simulink model "LANSwitch"  (R2022b)
settings: Solver=FixedStepAuto  StartTime=0.0  StopTime=10.0  FixedStep=1  RelTol=1e-3
libraries: simulink x34
settings Model: Creator=sadamu  LastModifiedBy=yuzehong
settings OptimizationCC: DefaultParameterBehavior=Inlined  BufferReuse=off  GlobalBufferReuse=off  ExpressionFolding=off  EnableMemcpy=off  PassReuseOutputArgsAs=Individual arguments  NoFixptDivByZeroProtection=on  EfficientFloat2IntCast=on  OptimizeDataStoreBuffers=off  BusAssignmentInplaceUpdate=off  OptimizationLevel=level0  EfficientTunableParamExpr=on
settings DebuggingCC: ParameterTunabilityLossMsg=error  AllowSymbolicDim=off
settings SFSimCC: MATLABDynamicMemAlloc=off
settings RTWCC: Description=Embedded Coder  SystemTargetFile=ert.tlc  GenCodeOnly=on  TemplateMakefile=ert_default_tmf
settings CodeAppCC: GenerateComments=off  IgnoreCustomStorageClasses=off  OperatorAnnotations=on  SimulinkDataObjDesc=on  SFDataObjDesc=on  SimulinkBlockComments=off
settings ERTTargetCC: TargetLangStandard=C99 (ISO)  GenerateSampleERTMain=on  CodeInterfacePackaging=Reusable function  InlinedParameterPlacement=NonHierarchical  ERTCustomFileTemplate=example_file_process.tlc
settings ConfigComp: CovMetricSettings=dcmwe  DVMaxProcessTime=3600  DVTestSuiteOptimization=Auto  DVDetectOutOfBounds=on  DVModelReferenceHarness=on

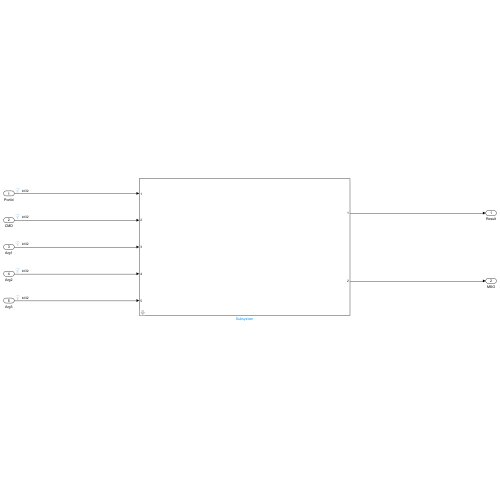
[thumbnail: Simulink's stored preview of the top-level diagram]
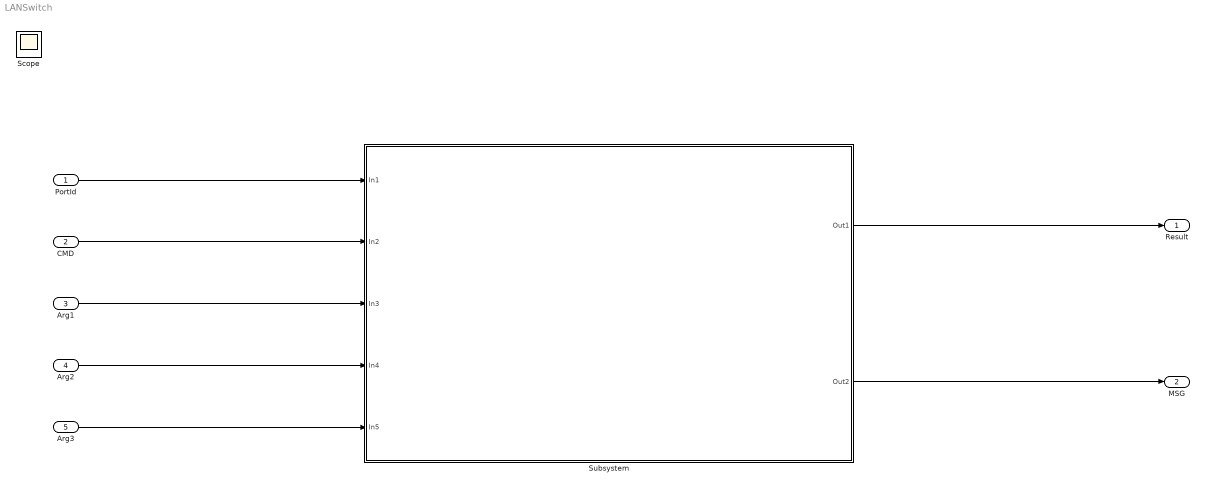
== system LANSwitch ==
  PortId : Inport  OutDataTypeStr=int32
  CMD : Inport  Port=2  OutDataTypeStr=int32
  Arg1 : Inport  Port=3  OutDataTypeStr=int32
  Arg2 : Inport  Port=4  OutDataTypeStr=int32
  Arg3 : Inport  Port=5  OutDataTypeStr=int32
  Subsystem : Subsystem  mask{POOL_SIZE=256}
      mask DialogControl ParameterGroupVar Prompt: 参数
  Result : Outport
  MSG : Outport  Port=2
  Scope : Scope
  wires:
  PortId/1 -> Subsystem/1(In1)
  CMD/1 -> Subsystem/2(In2)
  Arg1/1 -> Subsystem/3(In3)
  Arg2/1 -> Subsystem/4(In4)
  Arg3/1 -> Subsystem/5(In5)
  Subsystem/1(Out1) -> Result/1
  Subsystem/2(Out2) -> MSG/1

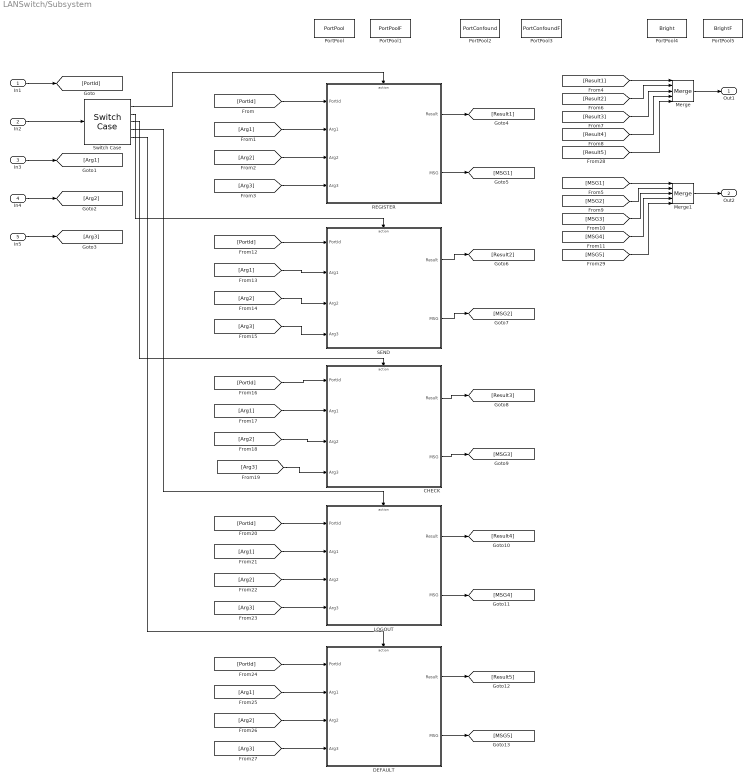
== system LANSwitch/Subsystem ==
  In1 : Inport
  In2 : Inport  Port=2
  In3 : Inport  Port=3
  In4 : Inport  Port=4
  In5 : Inport  Port=5
  CHECK : Subsystem  TreatAsAtomicUnit=on
  DEFAULT : Subsystem  TreatAsAtomicUnit=on
  LOGOUT : Subsystem  TreatAsAtomicUnit=on
  Merge : Merge  Inputs=5
  Merge1 : Merge  Inputs=5
  PortPool : DataStoreMemory  DataStoreName=PortPool  WriteAfterWriteMsg=warning  ShowAdditionalParam=off  OutDataTypeStr=int32  Dimensions=POOL_SIZE
  PortPool1 : DataStoreMemory  DataStoreName=PortPoolF  WriteAfterWriteMsg=warning  ShowAdditionalParam=off  OutDataTypeStr=int32  Dimensions=POOL_SIZE
  PortPool2 : DataStoreMemory  DataStoreName=PortConfound  WriteAfterWriteMsg=warning  ShowAdditionalParam=off  OutDataTypeStr=int32  Dimensions=POOL_SIZE
  PortPool3 : DataStoreMemory  DataStoreName=PortConfoundF  WriteAfterWriteMsg=warning  ShowAdditionalParam=off  OutDataTypeStr=int32  Dimensions=POOL_SIZE
  PortPool4 : DataStoreMemory  DataStoreName=Bright  WriteAfterWriteMsg=warning  ShowAdditionalParam=off  OutDataTypeStr=int32  Dimensions=POOL_SIZE
  PortPool5 : DataStoreMemory  DataStoreName=BrightF  WriteAfterWriteMsg=warning  ShowAdditionalParam=off  OutDataTypeStr=int32  Dimensions=POOL_SIZE
  REGISTER : Subsystem  TreatAsAtomicUnit=on
  SEND : Subsystem  TreatAsAtomicUnit=on
  Switch Case : SwitchCase  CaseConditions={10001, 10002, 10003, 10004}
  Out1 : Outport
  Out2 : Outport  Port=2
  wires:
  DEFAULT/1(Result) -> [Result5]
  REGISTER/1(Result) -> [Result1]
  In2/1 -> Switch Case/1
  [PortId] -> REGISTER/1(PortId)
  [Arg3] -> LOGOUT/4(Arg3)
  CHECK/1(Result) -> [Result3]
  [MSG4] -> Merge1/4
  [Result1] -> Merge/1
  [MSG1] -> Merge1/1
  LOGOUT/2(MSG) -> [MSG4]
  CHECK/2(MSG) -> [MSG3]
  REGISTER/2(MSG) -> [MSG1]
  [Result3] -> Merge/3
  [Arg3] -> SEND/4(Arg3)
  [Arg1] -> REGISTER/2(Arg1)
  [Result5] -> Merge/5
  [Result2] -> Merge/2
  [Result4] -> Merge/4
  [Arg2] -> SEND/3(Arg2)
  [MSG2] -> Merge1/2
  [Arg3] -> DEFAULT/4(Arg3)
  SEND/1(Result) -> [Result2]
  [Arg1] -> SEND/2(Arg1)
  [Arg2] -> REGISTER/3(Arg2)
  [MSG3] -> Merge1/3
  [Arg2] -> DEFAULT/3(Arg2)
  [PortId] -> CHECK/1(PortId)
  Switch Case/2 -> SEND/Action
  In4/1 -> [Arg2]
  Switch Case/5 -> DEFAULT/Action
  SEND/2(MSG) -> [MSG2]
  Switch Case/4 -> LOGOUT/Action
  [Arg2] -> CHECK/3(Arg2)
  [MSG5] -> Merge1/5
  [PortId] -> LOGOUT/1(PortId)
  In5/1 -> [Arg3]
  [Arg3] -> REGISTER/4(Arg3)
  [Arg1] -> DEFAULT/2(Arg1)
  [Arg2] -> LOGOUT/3(Arg2)
  DEFAULT/2(MSG) -> [MSG5]
  Switch Case/3 -> CHECK/Action
  [Arg1] -> CHECK/2(Arg1)
  [PortId] -> SEND/1(PortId)
  In1/1 -> [PortId]
  [Arg3] -> CHECK/4(Arg3)
  LOGOUT/1(Result) -> [Result4]
  Switch Case/1 -> REGISTER/Action
  Merge1/1 -> Out2/1
  [Arg1] -> LOGOUT/2(Arg1)
  [PortId] -> DEFAULT/1(PortId)
  In3/1 -> [Arg1]
  Merge/1 -> Out1/1

== system LANSwitch/Subsystem/CHECK ==
  PortId : Inport
  Arg1 : Inport  Port=2
  Arg2 : Inport  Port=3
  Arg3 : Inport  Port=4
  Action Port : ActionPort  ActionPortLabel=case [ 10003 ]:
  Compare To Constant : simulink/Logic and Bit Operations/Compare To Constant  relop===  const=0  OutDataTypeStr=boolean
  Error : Subsystem  TreatAsAtomicUnit=on
  Handle : Subsystem  TreatAsAtomicUnit=on
  If : If  IfExpression=u1 ~= 0
  Merge : Merge
  Merge1 : Merge
  Result : Outport
  MSG : Outport  Port=2
  wires:
  Arg1/1 -> Handle/2(Arg1)
  Arg2/1 -> Handle/3(Arg2)
  Arg3/1 -> Handle/4(Arg3)
  Merge/1 -> Result/1
  Error/2(MSG) -> Merge1/1
  If/1 -> Error/Action
  If/2 -> Handle/Action
  Merge1/1 -> MSG/1
  PortId/1 -> Handle/1(PortId), Compare To Constant/1
  Error/1(Result) -> Merge/1
  Handle/2(MSG) -> Merge1/2
  Handle/1(Result) -> Merge/2
  Compare To Constant/1 -> If/1

== system LANSwitch/Subsystem/DEFAULT ==
  PortId : Inport
  Arg1 : Inport  Port=2
  Arg2 : Inport  Port=3
  Arg3 : Inport  Port=4
  Action Port : ActionPort  ActionPortLabel=default:
  Constant : Constant  Value=-10002  OutDataTypeStr=int32
  Constant1 : Constant  Value=0  OutDataTypeStr=int32
  Terminator{,1..3} (4 alike) : Terminator
  Result : Outport
  MSG : Outport  Port=2
  wires:
  Constant/1 -> Result/1
  PortId/1 -> Terminator/1
  Arg1/1 -> Terminator1/1
  Arg2/1 -> Terminator2/1
  Arg3/1 -> Terminator3/1
  Constant1/1 -> MSG/1

== system LANSwitch/Subsystem/LOGOUT ==
  PortId : Inport
  Arg1 : Inport  Port=2
  Arg2 : Inport  Port=3
  Arg3 : Inport  Port=4
  Action Port : ActionPort  ActionPortLabel=case [ 10004 ]:
  Compare To Constant : simulink/Logic and Bit Operations/Compare To Constant  relop===  const=0  OutDataTypeStr=boolean
  Error : Subsystem  TreatAsAtomicUnit=on
  Handle : Subsystem  TreatAsAtomicUnit=on
  If : If  IfExpression=u1 ~= 0
  Merge : Merge
  Merge1 : Merge
  Result : Outport
  MSG : Outport  Port=2
  wires:
  PortId/1 -> Handle/1(PortId), Compare To Constant/1
  Compare To Constant/1 -> If/1
  Arg2/1 -> Handle/3(Arg2)
  Error/2(MSG) -> Merge1/1
  Arg1/1 -> Handle/2(Arg1)
  Handle/1(Result) -> Merge/2
  Merge1/1 -> MSG/1
  Error/1(Result) -> Merge/1
  Merge/1 -> Result/1
  If/1 -> Error/Action
  If/2 -> Handle/Action
  Arg3/1 -> Handle/4(Arg3)
  Handle/2(MSG) -> Merge1/2

== system LANSwitch/Subsystem/REGISTER ==
  PortId : Inport
  Arg1 : Inport  Port=2
  Arg2 : Inport  Port=3
  Arg3 : Inport  Port=4
  Action Port : ActionPort  ActionPortLabel=case [ 10001 ]:
  Compare To Constant : simulink/Logic and Bit Operations/Compare To Constant  relop===  const=0  OutDataTypeStr=boolean
  Error : Subsystem  TreatAsAtomicUnit=on
  Handle : Subsystem  TreatAsAtomicUnit=on
  If : If  IfExpression=u1 ~= 0
  Merge : Merge
  Merge1 : Merge
  Result : Outport
  MSG : Outport  Port=2
  wires:
  PortId/1 -> Handle/1(PortId), Compare To Constant/1
  Compare To Constant/1 -> If/1
  If/1 -> Error/Action
  If/2 -> Handle/Action
  Error/1(Result) -> Merge/1
  Handle/1(Result) -> Merge/2
  Merge/1 -> Result/1
  Merge1/1 -> MSG/1
  Error/2(MSG) -> Merge1/1
  Handle/2(MSG) -> Merge1/2
  Arg1/1 -> Handle/2(Arg1)
  Arg2/1 -> Handle/3(Arg2)
  Arg3/1 -> Handle/4(Arg3)

== system LANSwitch/Subsystem/SEND ==
  PortId : Inport
  Arg1 : Inport  Port=2
  Arg2 : Inport  Port=3
  Arg3 : Inport  Port=4
  Action Port : ActionPort  ActionPortLabel=case [ 10002 ]:
  Compare To Constant : simulink/Logic and Bit Operations/Compare To Constant  relop===  const=0  OutDataTypeStr=boolean
  Error : Subsystem  TreatAsAtomicUnit=on
  Handle : Subsystem  TreatAsAtomicUnit=on
  If : If  IfExpression=u1 ~= 0
  Merge : Merge
  Merge1 : Merge
  Result : Outport
  MSG : Outport  Port=2
  wires:
  Arg1/1 -> Handle/2(Arg1)
  Arg2/1 -> Handle/3(Arg2)
  Arg3/1 -> Handle/4(Arg3)
  Merge/1 -> Result/1
  Error/2(MSG) -> Merge1/1
  If/1 -> Error/Action
  If/2 -> Handle/Action
  Merge1/1 -> MSG/1
  PortId/1 -> Handle/1(PortId), Compare To Constant/1
  Error/1(Result) -> Merge/1
  Handle/2(MSG) -> Merge1/2
  Handle/1(Result) -> Merge/2
  Compare To Constant/1 -> If/1

== system LANSwitch/Subsystem/CHECK/Error ==
  Action Port : ActionPort  ActionPortLabel=if(u1 ~= 0)
  Constant : Constant  Value=-10001  OutDataTypeStr=int32
  Constant1 : Constant  Value=0  OutDataTypeStr=int32
  Result : Outport
  MSG : Outport  Port=2
  wires:
  Constant/1 -> Result/1
  Constant1/1 -> MSG/1

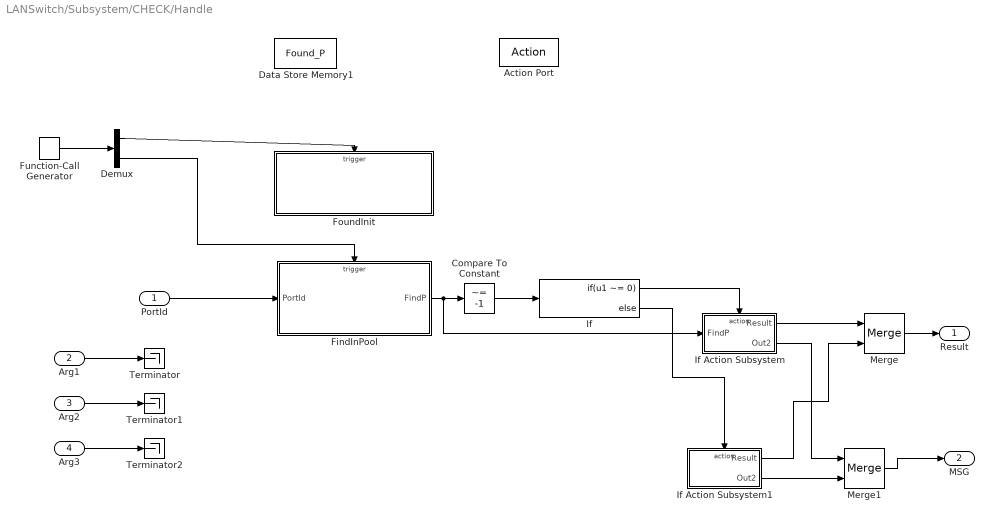
== system LANSwitch/Subsystem/CHECK/Handle ==
  PortId : Inport
  Arg1 : Inport  Port=2
  Arg2 : Inport  Port=3
  Arg3 : Inport  Port=4
  Action Port : ActionPort  ActionPortLabel=else
  Compare To Constant : simulink/Logic and Bit Operations/Compare To Constant  relop=~=  const=-1  OutDataTypeStr=boolean
  Data Store Memory1 : DataStoreMemory  DataStoreName=Found_P  WriteAfterWriteMsg=warning  InitialValue=-1  ShowAdditionalParam=off  OutDataTypeStr=int32
  Demux : Demux  Outputs=2
  FindInPool : Subsystem
  FoundInit : Subsystem
  Function-Call Generator : simulink/Ports & Subsystems/Function-Call Generator  sample_time=1  numberOfIterations=1  DisallowWideOutput=off
  If : If  IfExpression=u1 ~= 0
  If Action Subsystem : Subsystem  TreatAsAtomicUnit=on
  If Action Subsystem1 : Subsystem  TreatAsAtomicUnit=on
  Merge : Merge
  Merge1 : Merge
  Terminator : Terminator
  Terminator1 : Terminator
  Terminator2 : Terminator
  Result : Outport
  MSG : Outport  Port=2
  wires:
  Function-Call Generator/1 -> Demux/1
  Demux/1 -> FoundInit/Trigger
  Demux/2 -> FindInPool/Trigger
  PortId/1 -> FindInPool/1(PortId)
  Arg1/1 -> Terminator/1
  Arg2/1 -> Terminator1/1
  Arg3/1 -> Terminator2/1
  FindInPool/1(FindP) -> If Action Subsystem/1(FindP), Compare To Constant/1
  Compare To Constant/1 -> If/1
  If/1 -> If Action Subsystem/Action
  Merge/1 -> Result/1
  Merge1/1 -> MSG/1
  If Action Subsystem/1(Result) -> Merge/1
  If Action Subsystem/2(Out2) -> Merge1/1
  If Action Subsystem1/1(Result) -> Merge/2
  If Action Subsystem1/2(Out2) -> Merge1/2
  If/2 -> If Action Subsystem1/Action

== system LANSwitch/Subsystem/LOGOUT/Error ==
  Action Port : ActionPort  ActionPortLabel=if(u1 ~= 0)
  Constant : Constant  Value=-10001  OutDataTypeStr=int32
  Constant1 : Constant  Value=0  OutDataTypeStr=int32
  Result : Outport
  MSG : Outport  Port=2
  wires:
  Constant/1 -> Result/1
  Constant1/1 -> MSG/1

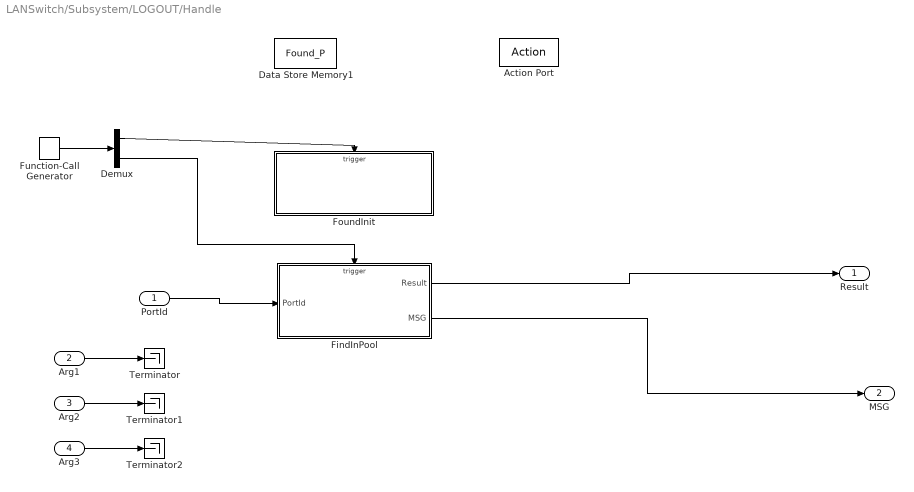
== system LANSwitch/Subsystem/LOGOUT/Handle ==
  PortId : Inport
  Arg1 : Inport  Port=2
  Arg2 : Inport  Port=3
  Arg3 : Inport  Port=4
  Action Port : ActionPort  ActionPortLabel=else
  Data Store Memory1 : DataStoreMemory  DataStoreName=Found_P  WriteAfterWriteMsg=warning  InitialValue=-1  ShowAdditionalParam=off  OutDataTypeStr=int32
  Demux : Demux  Outputs=2
  FindInPool : Subsystem
  FoundInit : Subsystem
  Function-Call Generator : simulink/Ports & Subsystems/Function-Call Generator  sample_time=1  numberOfIterations=1  DisallowWideOutput=off
  Terminator : Terminator
  Terminator1 : Terminator
  Terminator2 : Terminator
  Result : Outport
  MSG : Outport  Port=2
  wires:
  Function-Call Generator/1 -> Demux/1
  Demux/1 -> FoundInit/Trigger
  Demux/2 -> FindInPool/Trigger
  PortId/1 -> FindInPool/1(PortId)
  Arg1/1 -> Terminator/1
  Arg2/1 -> Terminator1/1
  Arg3/1 -> Terminator2/1
  FindInPool/1(Result) -> Result/1
  FindInPool/2(MSG) -> MSG/1

== system LANSwitch/Subsystem/REGISTER/Error ==
  Action Port : ActionPort  ActionPortLabel=if(u1 ~= 0)
  Constant : Constant  Value=-10001  OutDataTypeStr=int32
  Constant1 : Constant  Value=0  OutDataTypeStr=int32
  Result : Outport
  MSG : Outport  Port=2
  wires:
  Constant/1 -> Result/1
  Constant1/1 -> MSG/1

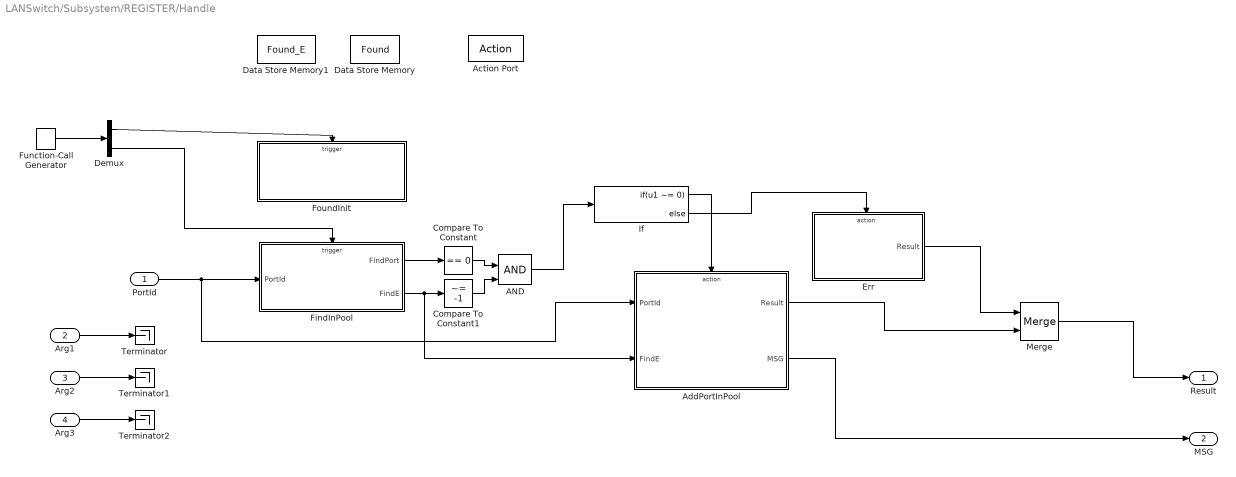
== system LANSwitch/Subsystem/REGISTER/Handle ==
  PortId : Inport
  Arg1 : Inport  Port=2
  Arg2 : Inport  Port=3
  Arg3 : Inport  Port=4
  Action Port : ActionPort  ActionPortLabel=else
  AND : Logic  IconShape=distinctive  AllPortsSameDT=off  OutDataTypeStr=boolean
  AddPortInPool : Subsystem  TreatAsAtomicUnit=on
  Compare To Constant : simulink/Logic and Bit Operations/Compare To Constant  relop===  const=0  OutDataTypeStr=boolean
  Compare To Constant1 : simulink/Logic and Bit Operations/Compare To Constant  relop=~=  const=-1  OutDataTypeStr=boolean
  Data Store Memory : DataStoreMemory  DataStoreName=Found  WriteAfterWriteMsg=warning  ShowAdditionalParam=off  OutDataTypeStr=boolean
  Data Store Memory1 : DataStoreMemory  DataStoreName=Found_E  WriteAfterWriteMsg=warning  InitialValue=-1  ShowAdditionalParam=off  OutDataTypeStr=int32
  Demux : Demux  Outputs=2
  Err : Subsystem  TreatAsAtomicUnit=on
  FindInPool : Subsystem
  FoundInit : Subsystem
  Function-Call Generator : simulink/Ports & Subsystems/Function-Call Generator  sample_time=1  numberOfIterations=1  DisallowWideOutput=off
  If : If  IfExpression=u1 ~= 0
  Merge : Merge
  Terminator : Terminator
  Terminator1 : Terminator
  Terminator2 : Terminator
  Result : Outport
  MSG : Outport  Port=2
  wires:
  Function-Call Generator/1 -> Demux/1
  Demux/1 -> FoundInit/Trigger
  Demux/2 -> FindInPool/Trigger
  PortId/1 -> FindInPool/1(PortId), AddPortInPool/1(PortId)
  AND/1 -> If/1
  Merge/1 -> Result/1
  Err/1(Result) -> Merge/1
  AddPortInPool/1(Result) -> Merge/2
  AddPortInPool/2(MSG) -> MSG/1
  Arg1/1 -> Terminator/1
  Arg2/1 -> Terminator1/1
  Arg3/1 -> Terminator2/1
  FindInPool/1(FindPort) -> Compare To Constant/1
  FindInPool/2(FindE) -> AddPortInPool/2(FindE), Compare To Constant1/1
  Compare To Constant/1 -> AND/1
  Compare To Constant1/1 -> AND/2
  If/2 -> Err/Action
  If/1 -> AddPortInPool/Action

== system LANSwitch/Subsystem/SEND/Error ==
  Action Port : ActionPort  ActionPortLabel=if(u1 ~= 0)
  Constant : Constant  Value=-10001  OutDataTypeStr=int32
  Constant1 : Constant  Value=0  OutDataTypeStr=int32
  Result : Outport
  MSG : Outport  Port=2
  wires:
  Constant/1 -> Result/1
  Constant1/1 -> MSG/1

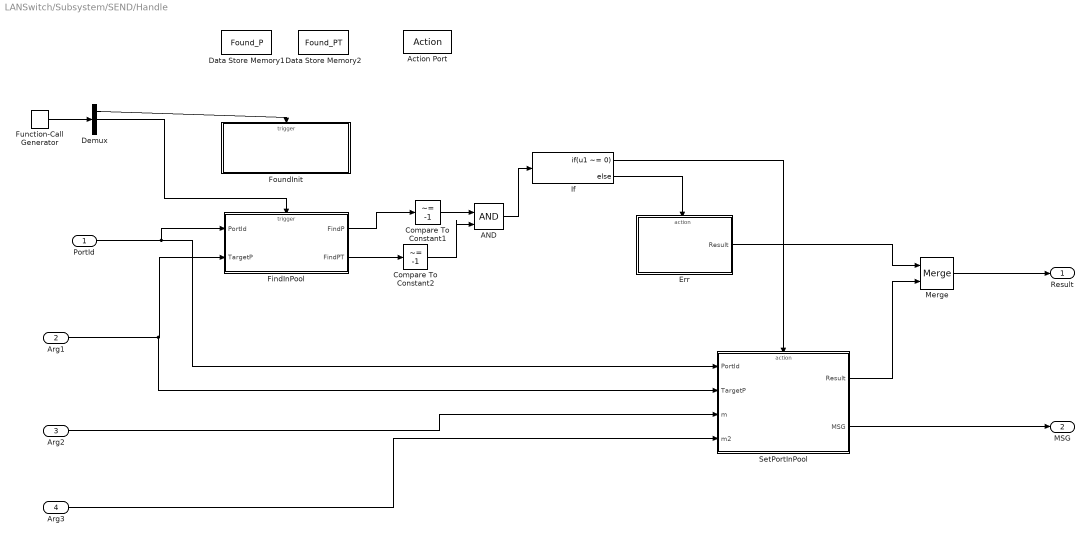
== system LANSwitch/Subsystem/SEND/Handle ==
  PortId : Inport
  Arg1 : Inport  Port=2
  Arg2 : Inport  Port=3
  Arg3 : Inport  Port=4
  Action Port : ActionPort  ActionPortLabel=else
  AND : Logic  IconShape=distinctive  AllPortsSameDT=off  OutDataTypeStr=boolean
  Compare To Constant1 : simulink/Logic and Bit Operations/Compare To Constant  relop=~=  const=-1  OutDataTypeStr=boolean
  Compare To Constant2 : simulink/Logic and Bit Operations/Compare To Constant  relop=~=  const=-1  OutDataTypeStr=boolean
  Data Store Memory1 : DataStoreMemory  DataStoreName=Found_P  WriteAfterWriteMsg=warning  InitialValue=-1  ShowAdditionalParam=off  OutDataTypeStr=int32
  Data Store Memory2 : DataStoreMemory  DataStoreName=Found_PT  WriteAfterWriteMsg=warning  InitialValue=-1  ShowAdditionalParam=off  OutDataTypeStr=int32
  Demux : Demux  Outputs=3
  Err : Subsystem  TreatAsAtomicUnit=on
  FindInPool : Subsystem
  FoundInit : Subsystem
  Function-Call Generator : simulink/Ports & Subsystems/Function-Call Generator  sample_time=1  numberOfIterations=1  DisallowWideOutput=off
  If : If  IfExpression=u1 ~= 0
  Merge : Merge
  SetPortInPool : Subsystem  TreatAsAtomicUnit=on
  Result : Outport
  MSG : Outport  Port=2
  wires:
  Function-Call Generator/1 -> Demux/1
  Demux/1 -> FoundInit/Trigger
  Demux/2 -> FindInPool/Trigger
  PortId/1 -> SetPortInPool/1(PortId), FindInPool/1(PortId)
  If/1 -> SetPortInPool/Action
  Merge/1 -> Result/1
  SetPortInPool/2(MSG) -> MSG/1
  Arg3/1 -> SetPortInPool/4(m2)
  FindInPool/1(FindP) -> Compare To Constant1/1
  Arg1/1 -> SetPortInPool/2(TargetP), FindInPool/2(TargetP)
  FindInPool/2(FindPT) -> Compare To Constant2/1
  Compare To Constant1/1 -> AND/1
  Compare To Constant2/1 -> AND/2
  AND/1 -> If/1
  If/2 -> Err/Action
  SetPortInPool/1(Result) -> Merge/2
  Err/1(Result) -> Merge/1
  Arg2/1 -> SetPortInPool/3(m)

== system LANSwitch/Subsystem/CHECK/Handle/FindInPool ==
  PortId : Inport
  function : TriggerPort  TriggerType=function-call  VariantControl=(inherit)
  FindPortInPool : Subsystem  TreatAsAtomicUnit=on
  FindP : Outport
  wires:
  PortId/1 -> FindPortInPool/1(PortId)
  FindPortInPool/1(Out1) -> FindP/1

== system LANSwitch/Subsystem/CHECK/Handle/FoundInit ==
  function : TriggerPort  TriggerType=function-call  VariantControl=(inherit)
  Constant1 : Constant  Value=-1  OutDataTypeStr=int32
  Data Store Write1 : DataStoreWrite  DataStoreName=Found_P  IndexOptions=Index vector (dialog)  Indices=1  OutputSizes=1
  wires:
  Constant1/1 -> Data Store Write1/1

== system LANSwitch/Subsystem/CHECK/Handle/If Action Subsystem ==
  FindP : Inport
  Action Port : ActionPort  ActionPortLabel=if(u1 ~= 0)
  Constant : Constant  OutDataTypeStr=int32
  Result : Outport
  Out2 : Outport  Port=2
  wires:
  FindP/1 -> Result/1
  Constant/1 -> Out2/1

== system LANSwitch/Subsystem/CHECK/Handle/If Action Subsystem1 ==
  Action Port : ActionPort  ActionPortLabel=else
  Constant : Constant  Value=-1  OutDataTypeStr=int32
  Constant1 : Constant  Value=-1  OutDataTypeStr=int32
  Result : Outport
  Out2 : Outport  Port=2
  wires:
  Constant/1 -> Out2/1
  Constant1/1 -> Result/1

== system LANSwitch/Subsystem/LOGOUT/Handle/FindInPool ==
  PortId : Inport
  function : TriggerPort  TriggerType=function-call  VariantControl=(inherit)
  Compare To Constant1 : simulink/Logic and Bit Operations/Compare To Constant  relop===  const=-1  OutDataTypeStr=uint8
  Err : Subsystem  TreatAsAtomicUnit=on
  FindPortInPool : Subsystem  TreatAsAtomicUnit=on
  If : If  IfExpression=u1 ~= 0
  Merge : Merge
  SetPortInPool : Subsystem  TreatAsAtomicUnit=on
  Result : Outport
  MSG : Outport  Port=2
  wires:
  SetPortInPool/2(MSG) -> MSG/1
  If/1 -> Err/Action
  PortId/1 -> SetPortInPool/1(PortId), FindPortInPool/1(PortId)
  FindPortInPool/1(Out1) -> Compare To Constant1/1
  Err/1(Result) -> Merge/1
  If/2 -> SetPortInPool/Action
  Compare To Constant1/1 -> If/1
  Merge/1 -> Result/1
  SetPortInPool/1(Result) -> Merge/2

== system LANSwitch/Subsystem/LOGOUT/Handle/FoundInit ==
  function : TriggerPort  TriggerType=function-call  VariantControl=(inherit)
  Constant1 : Constant  Value=-1  OutDataTypeStr=int32
  Data Store Write1 : DataStoreWrite  DataStoreName=Found_P  IndexOptions=Index vector (dialog)  Indices=1  OutputSizes=1
  wires:
  Constant1/1 -> Data Store Write1/1

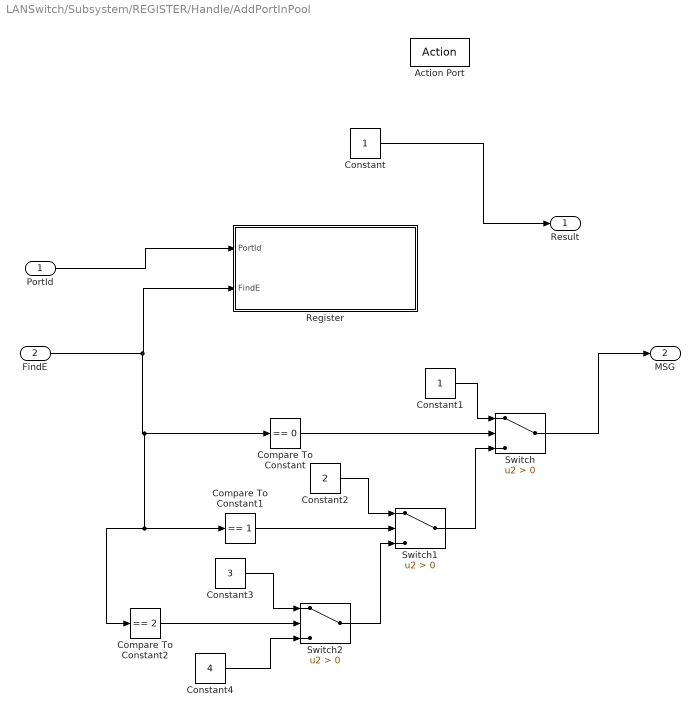
== system LANSwitch/Subsystem/REGISTER/Handle/AddPortInPool ==
  PortId : Inport
  FindE : Inport  Port=2
  Action Port : ActionPort  ActionPortLabel=if(u1 ~= 0)
  Compare To Constant : simulink/Logic and Bit Operations/Compare To Constant  relop===  const=0  OutDataTypeStr=boolean
  Compare To Constant1 : simulink/Logic and Bit Operations/Compare To Constant  relop===  const=1  OutDataTypeStr=boolean
  Compare To Constant2 : simulink/Logic and Bit Operations/Compare To Constant  relop===  const=2  OutDataTypeStr=boolean
  Constant : Constant  OutDataTypeStr=int32
  Constant1 : Constant  OutDataTypeStr=int32
  Constant2 : Constant  Value=2  OutDataTypeStr=int32
  Constant3 : Constant  Value=3  OutDataTypeStr=int32
  Constant4 : Constant  Value=4  OutDataTypeStr=int32
  Register : Subsystem  TreatAsAtomicUnit=on
  Switch : Switch  Criteria=u2 > Threshold  SaturateOnIntegerOverflow=off  InputSameDT=off
  Switch1 : Switch  Criteria=u2 > Threshold  SaturateOnIntegerOverflow=off  InputSameDT=off
  Switch2 : Switch  Criteria=u2 > Threshold  SaturateOnIntegerOverflow=off  InputSameDT=off
  Result : Outport
  MSG : Outport  Port=2
  wires:
  PortId/1 -> Register/1(PortId)
  FindE/1 -> Compare To Constant2/1, Compare To Constant1/1, Compare To Constant/1, Register/2(FindE)
  Constant/1 -> Result/1
  Compare To Constant/1 -> Switch/2
  Constant1/1 -> Switch/1
  Constant2/1 -> Switch1/1
  Compare To Constant1/1 -> Switch1/2
  Switch1/1 -> Switch/3
  Compare To Constant2/1 -> Switch2/2
  Switch2/1 -> Switch1/3
  Constant3/1 -> Switch2/1
  Constant4/1 -> Switch2/3
  Switch/1 -> MSG/1

== system LANSwitch/Subsystem/REGISTER/Handle/Err ==
  Action Port : ActionPort  ActionPortLabel=else
  Constant : Constant  Value=-10004  OutDataTypeStr=int32
  Result : Outport
  wires:
  Constant/1 -> Result/1

== system LANSwitch/Subsystem/REGISTER/Handle/FindInPool ==
  PortId : Inport
  function : TriggerPort  TriggerType=function-call  VariantControl=(inherit)
  FindEmptyInPool : Subsystem  TreatAsAtomicUnit=on
  FindPortInPool : Subsystem  TreatAsAtomicUnit=on
  FindPort : Outport
  FindE : Outport  Port=2
  wires:
  FindPortInPool/1(Out1) -> FindPort/1
  PortId/1 -> FindPortInPool/1(PortId)
  FindEmptyInPool/1(Out1) -> FindE/1

== system LANSwitch/Subsystem/REGISTER/Handle/FoundInit ==
  function : TriggerPort  TriggerType=function-call  VariantControl=(inherit)
  Constant : Constant  Value=0  OutDataTypeStr=boolean
  Constant1 : Constant  Value=-1  OutDataTypeStr=int32
  Data Store Write : DataStoreWrite  DataStoreName=Found  IndexOptions=Index vector (dialog)  Indices=1  OutputSizes=1
  Data Store Write1 : DataStoreWrite  DataStoreName=Found_E  IndexOptions=Index vector (dialog)  Indices=1  OutputSizes=1
  wires:
  Constant/1 -> Data Store Write/1
  Constant1/1 -> Data Store Write1/1

== system LANSwitch/Subsystem/SEND/Handle/Err ==
  Action Port : ActionPort  ActionPortLabel=else
  Constant : Constant  Value=-10003  OutDataTypeStr=int32
  Result : Outport
  wires:
  Constant/1 -> Result/1

== system LANSwitch/Subsystem/SEND/Handle/FindInPool ==
  PortId : Inport
  TargetP : Inport  Port=2
  function : TriggerPort  TriggerType=function-call  VariantControl=(inherit)
  FindPortInPool : Subsystem  TreatAsAtomicUnit=on
  FindPortTInPool : Subsystem  TreatAsAtomicUnit=on
  FindP : Outport
  FindPT : Outport  Port=2
  wires:
  PortId/1 -> FindPortInPool/1(PortId)
  FindPortInPool/1(Out1) -> FindP/1
  TargetP/1 -> FindPortTInPool/1(PortId)
  FindPortTInPool/1(Out1) -> FindPT/1

== system LANSwitch/Subsystem/SEND/Handle/FoundInit ==
  function : TriggerPort  TriggerType=function-call  VariantControl=(inherit)
  Constant1 : Constant  Value=-1  OutDataTypeStr=int32
  Constant2 : Constant  Value=-1  OutDataTypeStr=int32
  Data Store Write1 : DataStoreWrite  DataStoreName=Found_P  IndexOptions=Index vector (dialog)  Indices=1  OutputSizes=1
  Data Store Write2 : DataStoreWrite  DataStoreName=Found_PT  IndexOptions=Index vector (dialog)  Indices=1  OutputSizes=1
  wires:
  Constant1/1 -> Data Store Write1/1
  Constant2/1 -> Data Store Write2/1

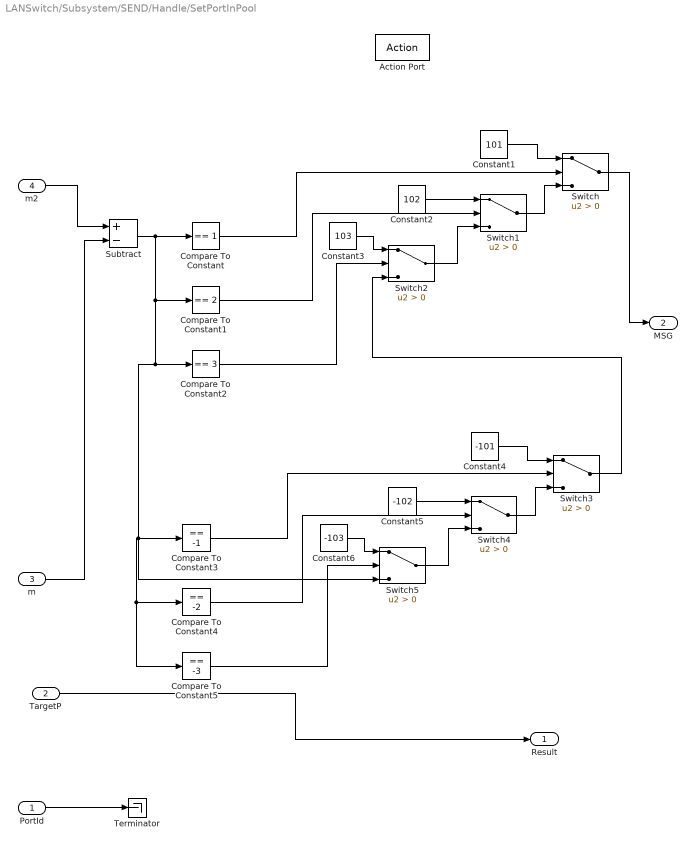
== system LANSwitch/Subsystem/SEND/Handle/SetPortInPool ==
  PortId : Inport
  TargetP : Inport  Port=2
  m : Inport  Port=3
  m2 : Inport  Port=4
  Action Port : ActionPort  ActionPortLabel=if(u1 ~= 0)
  Compare To Constant : simulink/Logic and Bit Operations/Compare To Constant  relop===  const=1  OutDataTypeStr=boolean
  Compare To Constant1 : simulink/Logic and Bit Operations/Compare To Constant  relop===  const=2  OutDataTypeStr=boolean
  Compare To Constant2 : simulink/Logic and Bit Operations/Compare To Constant  relop===  const=3  OutDataTypeStr=boolean
  Compare To Constant3 : simulink/Logic and Bit Operations/Compare To Constant  relop===  const=-1  OutDataTypeStr=boolean
  Compare To Constant4 : simulink/Logic and Bit Operations/Compare To Constant  relop===  const=-2  OutDataTypeStr=boolean
  Compare To Constant5 : simulink/Logic and Bit Operations/Compare To Constant  relop===  const=-3  OutDataTypeStr=boolean
  Constant1 : Constant  Value=101  OutDataTypeStr=int32
  Constant2 : Constant  Value=102  OutDataTypeStr=int32
  Constant3 : Constant  Value=103  OutDataTypeStr=int32
  Constant4 : Constant  Value=-101  OutDataTypeStr=int32
  Constant5 : Constant  Value=-102  OutDataTypeStr=int32
  Constant6 : Constant  Value=-103  OutDataTypeStr=int32
  Subtract : Sum  Inputs=+-
  Switch{,1..5} (6 alike) : Switch  Criteria=u2 > Threshold  SaturateOnIntegerOverflow=off  InputSameDT=off
  Terminator : Terminator
  Result : Outport
  MSG : Outport  Port=2
  wires:
  Compare To Constant/1 -> Switch/2
  Constant1/1 -> Switch/1
  Compare To Constant1/1 -> Switch1/2
  Constant2/1 -> Switch1/1
  Switch1/1 -> Switch/3
  Constant3/1 -> Switch2/1
  Switch2/1 -> Switch1/3
  Compare To Constant2/1 -> Switch2/2
  Constant4/1 -> Switch3/1
  Constant6/1 -> Switch5/1
  Constant5/1 -> Switch4/1
  Compare To Constant4/1 -> Switch4/2
  Compare To Constant5/1 -> Switch5/2
  Switch4/1 -> Switch3/3
  Subtract/1 -> Switch5/3, Compare To Constant5/1, Compare To Constant4/1, Compare To Constant3/1, Compare To Constant2/1, Compare To Constant1/1, Compare To Constant/1
  Compare To Constant3/1 -> Switch3/2
  Switch5/1 -> Switch4/3
  Switch3/1 -> Switch2/3
  Switch/1 -> MSG/1
  m/1 -> Subtract/2
  TargetP/1 -> Result/1
  m2/1 -> Subtract/1
  PortId/1 -> Terminator/1

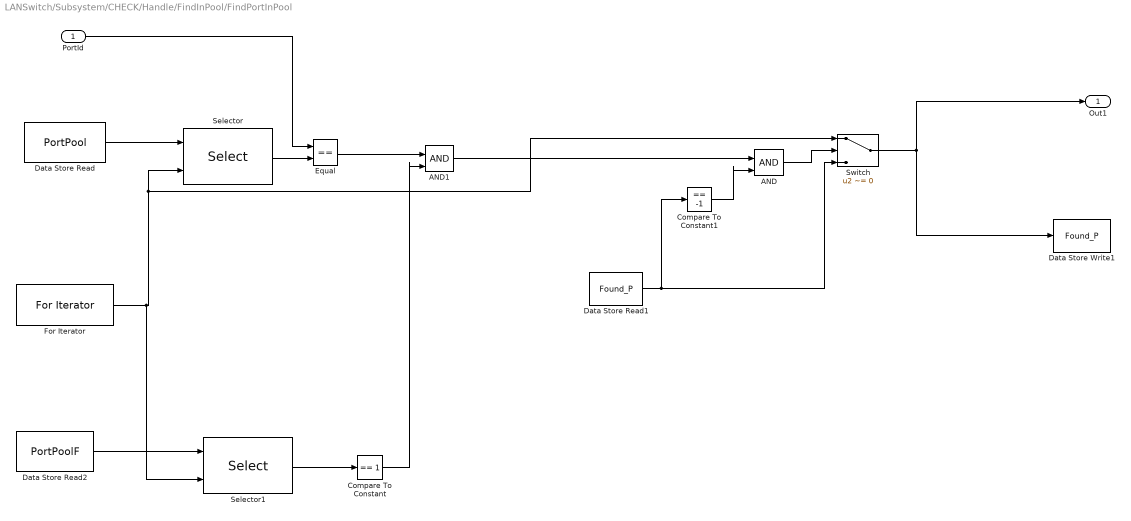
== system LANSwitch/Subsystem/CHECK/Handle/FindInPool/FindPortInPool ==
  PortId : Inport
  AND : Logic  IconShape=distinctive  AllPortsSameDT=off  OutDataTypeStr=boolean
  AND1 : Logic  IconShape=distinctive  AllPortsSameDT=off  OutDataTypeStr=boolean
  Compare To Constant : simulink/Logic and Bit Operations/Compare To Constant  relop===  const=1  OutDataTypeStr=boolean
  Compare To Constant1 : simulink/Logic and Bit Operations/Compare To Constant  relop===  const=-1  OutDataTypeStr=boolean
  Data Store Read : DataStoreRead  DataStoreName=PortPool  IndexOptions=Index vector (dialog)  Indices=1  OutputSizes=1
  Data Store Read1 : DataStoreRead  DataStoreName=Found_P  IndexOptions=Index vector (dialog)  Indices=1  OutputSizes=1
  Data Store Read2 : DataStoreRead  DataStoreName=PortPoolF  IndexOptions=Index vector (dialog)  Indices=1  OutputSizes=1
  Data Store Write1 : DataStoreWrite  DataStoreName=Found_P  IndexOptions=Index vector (dialog)  Indices=1  OutputSizes=1
  Equal : RelationalOperator  Operator===  OutDataTypeStr=boolean  RndMeth=Simplest  InputSameDT=off
  For Iterator : ForIterator  IterationLimit=POOL_SIZE  IndexMode=Zero-based
  Selector : Selector  IndexMode=Zero-based  InputPortWidth=POOL_SIZE  IndexOptions=Index vector (port)  Indices=[1 3]  OutputSizes=1
  Selector1 : Selector  IndexMode=Zero-based  InputPortWidth=POOL_SIZE  IndexOptions=Index vector (port)  Indices=[1 3]  OutputSizes=1
  Switch : Switch  Criteria=u2 ~= 0  SaturateOnIntegerOverflow=off  InputSameDT=off
  Out1 : Outport
  wires:
  Data Store Read/1 -> Selector/1
  Selector/1 -> Equal/2
  Equal/1 -> AND1/1
  Switch/1 -> Data Store Write1/1, Out1/1
  Data Store Read1/1 -> Compare To Constant1/1, Switch/3
  Compare To Constant1/1 -> AND/2
  AND/1 -> Switch/2
  PortId/1 -> Equal/1
  Compare To Constant/1 -> AND1/2
  Data Store Read2/1 -> Selector1/1
  For Iterator/1 -> Selector1/2, Switch/1, Selector/2
  Selector1/1 -> Compare To Constant/1
  AND1/1 -> AND/1

== system LANSwitch/Subsystem/LOGOUT/Handle/FindInPool/Err ==
  Action Port : ActionPort  ActionPortLabel=if(u1 ~= 0)
  Constant : Constant  Value=-10003  OutDataTypeStr=int32
  Result : Outport
  wires:
  Constant/1 -> Result/1

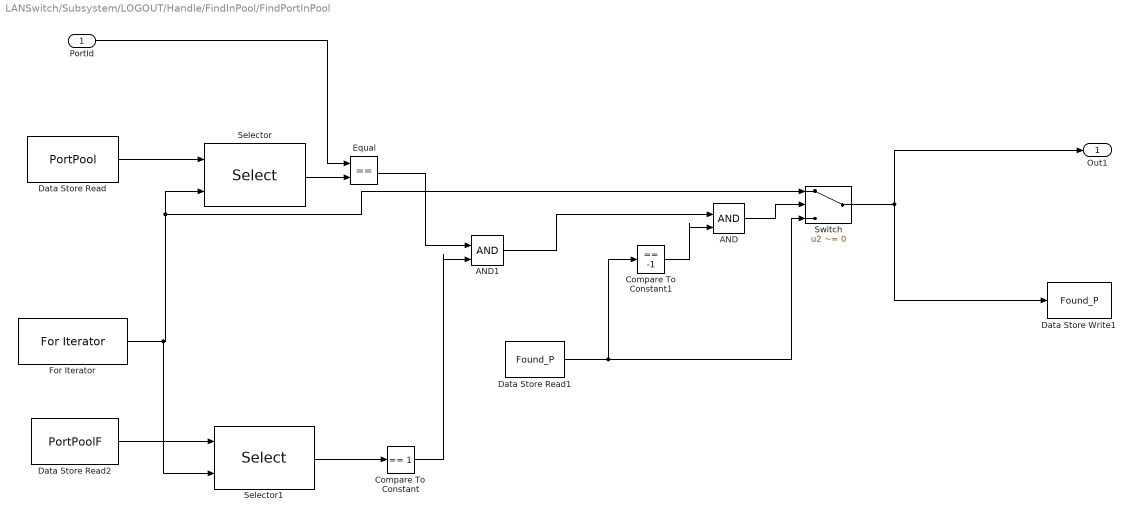
== system LANSwitch/Subsystem/LOGOUT/Handle/FindInPool/FindPortInPool ==
  PortId : Inport
  AND : Logic  IconShape=distinctive  AllPortsSameDT=off  OutDataTypeStr=boolean
  AND1 : Logic  IconShape=distinctive  AllPortsSameDT=off  OutDataTypeStr=boolean
  Compare To Constant : simulink/Logic and Bit Operations/Compare To Constant  relop===  const=1  OutDataTypeStr=boolean
  Compare To Constant1 : simulink/Logic and Bit Operations/Compare To Constant  relop===  const=-1  OutDataTypeStr=boolean
  Data Store Read : DataStoreRead  DataStoreName=PortPool  IndexOptions=Index vector (dialog)  Indices=1  OutputSizes=1
  Data Store Read1 : DataStoreRead  DataStoreName=Found_P  IndexOptions=Index vector (dialog)  Indices=1  OutputSizes=1
  Data Store Read2 : DataStoreRead  DataStoreName=PortPoolF  IndexOptions=Index vector (dialog)  Indices=1  OutputSizes=1
  Data Store Write1 : DataStoreWrite  DataStoreName=Found_P  IndexOptions=Index vector (dialog)  Indices=1  OutputSizes=1
  Equal : RelationalOperator  Operator===  OutDataTypeStr=boolean  RndMeth=Simplest  InputSameDT=off
  For Iterator : ForIterator  IterationLimit=POOL_SIZE  IndexMode=Zero-based
  Selector : Selector  IndexMode=Zero-based  InputPortWidth=POOL_SIZE  IndexOptions=Index vector (port)  Indices=[1 3]  OutputSizes=1
  Selector1 : Selector  IndexMode=Zero-based  InputPortWidth=POOL_SIZE  IndexOptions=Index vector (port)  Indices=[1 3]  OutputSizes=1
  Switch : Switch  Criteria=u2 ~= 0  SaturateOnIntegerOverflow=off  InputSameDT=off
  Out1 : Outport
  wires:
  Data Store Read/1 -> Selector/1
  Selector/1 -> Equal/2
  Equal/1 -> AND1/1
  Switch/1 -> Data Store Write1/1, Out1/1
  Data Store Read1/1 -> Compare To Constant1/1, Switch/3
  Compare To Constant1/1 -> AND/2
  AND/1 -> Switch/2
  PortId/1 -> Equal/1
  Compare To Constant/1 -> AND1/2
  Data Store Read2/1 -> Selector1/1
  For Iterator/1 -> Selector1/2, Switch/1, Selector/2
  Selector1/1 -> Compare To Constant/1
  AND1/1 -> AND/1

== system LANSwitch/Subsystem/LOGOUT/Handle/FindInPool/SetPortInPool ==
  PortId : Inport
  Action Port : ActionPort  ActionPortLabel=else
  Constant : Constant  OutDataTypeStr=int32
  LOGOUT : Subsystem  TreatAsAtomicUnit=on
  Result : Outport
  MSG : Outport  Port=2
  wires:
  PortId/1 -> Result/1, LOGOUT/1(FindP)
  Constant/1 -> MSG/1

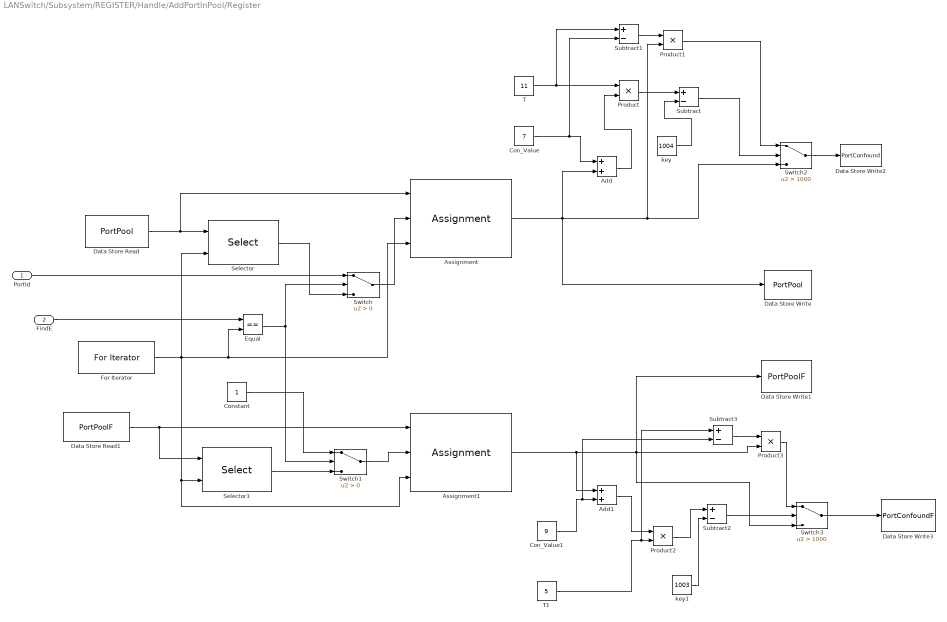
== system LANSwitch/Subsystem/REGISTER/Handle/AddPortInPool/Register ==
  PortId : Inport
  FindE : Inport  Port=2
  Add : Sum
  Add1 : Sum
  Assignment : Assignment  IndexMode=Zero-based  DiagnosticForDimensions=Warning  IndexOptions=Index vector (port)  Indices=1  OutputSizes=1
  Assignment1 : Assignment  IndexMode=Zero-based  DiagnosticForDimensions=Warning  IndexOptions=Index vector (port)  Indices=1  OutputSizes=1
  Con_Value : Constant  Value=7  OutDataTypeStr=int32
  Con_Value1 : Constant  Value=9  OutDataTypeStr=int32
  Constant : Constant  OutDataTypeStr=int32
  Data Store Read : DataStoreRead  DataStoreName=PortPool  IndexOptions=Index vector (dialog)  Indices=1  OutputSizes=1
  Data Store Read1 : DataStoreRead  DataStoreName=PortPoolF  IndexOptions=Index vector (dialog)  Indices=1  OutputSizes=1
  Data Store Write : DataStoreWrite  DataStoreName=PortPool  IndexOptions=Index vector (dialog)  Indices=1  OutputSizes=1
  Data Store Write1 : DataStoreWrite  DataStoreName=PortPoolF  IndexOptions=Index vector (dialog)  Indices=1  OutputSizes=1
  Data Store Write2 : DataStoreWrite  DataStoreName=PortConfound  IndexOptions=Index vector (dialog)  Indices=1  OutputSizes=1
  Data Store Write3 : DataStoreWrite  DataStoreName=PortConfoundF  IndexOptions=Index vector (dialog)  Indices=1  OutputSizes=1
  Equal : RelationalOperator  Operator===  OutDataTypeStr=boolean  RndMeth=Simplest  InputSameDT=off
  For Iterator : ForIterator  IterationLimit=POOL_SIZE  IndexMode=Zero-based
  Product{,1..3} (4 alike) : Product  OutDataTypeStr=int32
  Selector : Selector  IndexMode=Zero-based  InputPortWidth=POOL_SIZE  IndexOptions=Index vector (port)  Indices=[1 3]  OutputSizes=1
  Selector1 : Selector  IndexMode=Zero-based  InputPortWidth=POOL_SIZE  IndexOptions=Index vector (port)  Indices=[1 3]  OutputSizes=1
  Subtract : Sum  Inputs=+-  OutDataTypeStr=int32
  Subtract1 : Sum  Inputs=+-
  Subtract2 : Sum  Inputs=+-  OutDataTypeStr=int32
  Subtract3 : Sum  Inputs=+-  OutDataTypeStr=int32
  Switch : Switch  Criteria=u2 > Threshold  SaturateOnIntegerOverflow=off  InputSameDT=off
  Switch1 : Switch  Criteria=u2 > Threshold  SaturateOnIntegerOverflow=off  InputSameDT=off
  Switch2 : Switch  Criteria=u2 > Threshold  Threshold=1000  SaturateOnIntegerOverflow=off  InputSameDT=off
  Switch3 : Switch  Criteria=u2 > Threshold  Threshold=1000  SaturateOnIntegerOverflow=off  InputSameDT=off
  T : Constant  Value=11  OutDataTypeStr=int32
  T1 : Constant  Value=5
  key : Constant  Value=1004  OutDataTypeStr=int32
  key1 : Constant  Value=1003
  wires:
  For Iterator/1 -> Assignment1/3, Selector1/2, Selector/2, Assignment/3, Equal/2
  Data Store Read/1 -> Assignment/1, Selector/1
  FindE/1 -> Equal/1
  Equal/1 -> Switch1/2, Switch/2
  PortId/1 -> Switch/1
  Switch/1 -> Assignment/2
  Selector/1 -> Switch/3
  Assignment/1 -> Product1/2, Switch2/3, Add/2, Data Store Write/1
  Data Store Read1/1 -> Selector1/1, Assignment1/1
  Constant/1 -> Switch1/1
  Selector1/1 -> Switch1/3
  Switch1/1 -> Assignment1/2
  Assignment1/1 -> Add1/1, Product3/2, Switch3/3, Data Store Write1/1
  Switch2/1 -> Data Store Write2/1
  Con_Value/1 -> Subtract1/2, Add/1
  Add/1 -> Product/2
  T/1 -> Subtract1/1, Product/1
  Product/1 -> Subtract/1
  key/1 -> Subtract/2
  Subtract/1 -> Switch2/2
  Subtract1/1 -> Product1/1
  Product1/1 -> Switch2/1
  Con_Value1/1 -> Subtract3/2, Add1/2
  Add1/1 -> Product2/1
  T1/1 -> Subtract3/1, Product2/2
  Product2/1 -> Subtract2/1
  key1/1 -> Subtract2/2
  Subtract2/1 -> Switch3/2
  Switch3/1 -> Data Store Write3/1
  Subtract3/1 -> Product3/1
  Product3/1 -> Switch3/1

== system LANSwitch/Subsystem/REGISTER/Handle/FindInPool/FindEmptyInPool ==
  AND : Logic  IconShape=distinctive  AllPortsSameDT=off  OutDataTypeStr=boolean
  Compare To Constant1 : simulink/Logic and Bit Operations/Compare To Constant  relop===  const=-1  OutDataTypeStr=boolean
  Compare To Constant2 : simulink/Logic and Bit Operations/Compare To Constant  relop===  const=0  OutDataTypeStr=boolean
  Data Store Read1 : DataStoreRead  DataStoreName=Found_E  IndexOptions=Index vector (dialog)  Indices=1  OutputSizes=1
  Data Store Read2 : DataStoreRead  DataStoreName=PortPoolF  IndexOptions=Index vector (dialog)  Indices=1  OutputSizes=1
  Data Store Write1 : DataStoreWrite  DataStoreName=Found_E  IndexOptions=Index vector (dialog)  Indices=1  OutputSizes=1
  For Iterator : ForIterator  IterationLimit=POOL_SIZE  IndexMode=Zero-based
  Selector1 : Selector  IndexMode=Zero-based  InputPortWidth=POOL_SIZE  IndexOptions=Index vector (port)  Indices=[1 3]  OutputSizes=1
  Switch : Switch  Criteria=u2 ~= 0  SaturateOnIntegerOverflow=off  InputSameDT=off
  Out1 : Outport
  wires:
  Switch/1 -> Data Store Write1/1, Out1/1
  Data Store Read1/1 -> Compare To Constant1/1, Switch/3
  Compare To Constant1/1 -> AND/2
  AND/1 -> Switch/2
  For Iterator/1 -> Selector1/2, Switch/1
  Selector1/1 -> Compare To Constant2/1
  Data Store Read2/1 -> Selector1/1
  Compare To Constant2/1 -> AND/1

== system LANSwitch/Subsystem/REGISTER/Handle/FindInPool/FindPortInPool ==
  PortId : Inport
  AND : Logic  IconShape=distinctive  AllPortsSameDT=off  OutDataTypeStr=boolean
  Compare To Constant : simulink/Logic and Bit Operations/Compare To Constant  relop===  const=1  OutDataTypeStr=boolean
  Constant : Constant  OutDataTypeStr=boolean
  Data Store Read : DataStoreRead  DataStoreName=PortPool  IndexOptions=Index vector (dialog)  Indices=1  OutputSizes=1
  Data Store Read1 : DataStoreRead  DataStoreName=Found  IndexOptions=Index vector (dialog)  Indices=1  OutputSizes=1
  Data Store Read2 : DataStoreRead  DataStoreName=PortPoolF  IndexOptions=Index vector (dialog)  Indices=1  OutputSizes=1
  Data Store Write1 : DataStoreWrite  DataStoreName=Found  IndexOptions=Index vector (dialog)  Indices=1  OutputSizes=1
  Equal : RelationalOperator  Operator===  OutDataTypeStr=boolean  RndMeth=Simplest  InputSameDT=off
  For Iterator : ForIterator  IterationLimit=POOL_SIZE  IndexMode=Zero-based
  Selector : Selector  IndexMode=Zero-based  InputPortWidth=POOL_SIZE  IndexOptions=Index vector (port)  Indices=[1 3]  OutputSizes=1
  Selector1 : Selector  IndexMode=Zero-based  InputPortWidth=POOL_SIZE  IndexOptions=Index vector (port)  Indices=[1 3]  OutputSizes=1
  Switch : Switch  Criteria=u2 ~= 0  SaturateOnIntegerOverflow=off  InputSameDT=off
  Out1 : Outport
  wires:
  For Iterator/1 -> Selector1/2, Selector/2
  Data Store Read/1 -> Selector/1
  Selector/1 -> Equal/1
  PortId/1 -> Equal/2
  Equal/1 -> AND/1
  Constant/1 -> Switch/1
  Switch/1 -> Out1/1, Data Store Write1/1
  Data Store Read1/1 -> Switch/3
  Data Store Read2/1 -> Selector1/1
  Selector1/1 -> Compare To Constant/1
  Compare To Constant/1 -> AND/2
  AND/1 -> Switch/2

== system LANSwitch/Subsystem/SEND/Handle/FindInPool/FindPortInPool ==
  PortId : Inport
  AND : Logic  IconShape=distinctive  AllPortsSameDT=off  OutDataTypeStr=boolean
  AND1 : Logic  IconShape=distinctive  AllPortsSameDT=off  OutDataTypeStr=boolean
  Compare To Constant : simulink/Logic and Bit Operations/Compare To Constant  relop===  const=1  OutDataTypeStr=boolean
  Compare To Constant1 : simulink/Logic and Bit Operations/Compare To Constant  relop===  const=-1  OutDataTypeStr=boolean
  Data Store Read : DataStoreRead  DataStoreName=PortPool  IndexOptions=Index vector (dialog)  Indices=1  OutputSizes=1
  Data Store Read1 : DataStoreRead  DataStoreName=Found_P  IndexOptions=Index vector (dialog)  Indices=1  OutputSizes=1
  Data Store Read2 : DataStoreRead  DataStoreName=PortPoolF  IndexOptions=Index vector (dialog)  Indices=1  OutputSizes=1
  Data Store Write1 : DataStoreWrite  DataStoreName=Found_P  IndexOptions=Index vector (dialog)  Indices=1  OutputSizes=1
  Equal : RelationalOperator  Operator===  OutDataTypeStr=boolean  RndMeth=Simplest  InputSameDT=off
  For Iterator : ForIterator  IterationLimit=POOL_SIZE  IndexMode=Zero-based
  Selector : Selector  IndexMode=Zero-based  InputPortWidth=POOL_SIZE  IndexOptions=Index vector (port)  Indices=[1 3]  OutputSizes=1
  Selector1 : Selector  IndexMode=Zero-based  InputPortWidth=POOL_SIZE  IndexOptions=Index vector (port)  Indices=[1 3]  OutputSizes=1
  Switch : Switch  Criteria=u2 ~= 0  SaturateOnIntegerOverflow=off  InputSameDT=off
  Out1 : Outport
  wires:
  Data Store Read/1 -> Selector/1
  Selector/1 -> Equal/2
  Equal/1 -> AND1/1
  Switch/1 -> Data Store Write1/1, Out1/1
  Data Store Read1/1 -> Compare To Constant1/1, Switch/3
  Compare To Constant1/1 -> AND/2
  AND/1 -> Switch/2
  For Iterator/1 -> Selector1/2, Selector/2, Switch/1
  Selector1/1 -> Compare To Constant/1
  Data Store Read2/1 -> Selector1/1
  Compare To Constant/1 -> AND1/2
  AND1/1 -> AND/1
  PortId/1 -> Equal/1

== system LANSwitch/Subsystem/SEND/Handle/FindInPool/FindPortTInPool ==
  PortId : Inport
  AND : Logic  IconShape=distinctive  AllPortsSameDT=off  OutDataTypeStr=boolean
  AND1 : Logic  IconShape=distinctive  AllPortsSameDT=off  OutDataTypeStr=boolean
  Compare To Constant : simulink/Logic and Bit Operations/Compare To Constant  relop===  const=1  OutDataTypeStr=boolean
  Compare To Constant1 : simulink/Logic and Bit Operations/Compare To Constant  relop===  const=-1  OutDataTypeStr=boolean
  Data Store Read : DataStoreRead  DataStoreName=PortPool  IndexOptions=Index vector (dialog)  Indices=1  OutputSizes=1
  Data Store Read1 : DataStoreRead  DataStoreName=Found_PT  IndexOptions=Index vector (dialog)  Indices=1  OutputSizes=1
  Data Store Read2 : DataStoreRead  DataStoreName=PortPoolF  IndexOptions=Index vector (dialog)  Indices=1  OutputSizes=1
  Data Store Write1 : DataStoreWrite  DataStoreName=Found_PT  IndexOptions=Index vector (dialog)  Indices=1  OutputSizes=1
  Equal : RelationalOperator  Operator===  OutDataTypeStr=boolean  RndMeth=Simplest  InputSameDT=off
  For Iterator : ForIterator  IterationLimit=POOL_SIZE  IndexMode=Zero-based
  Selector : Selector  IndexMode=Zero-based  InputPortWidth=POOL_SIZE  IndexOptions=Index vector (port)  Indices=[1 3]  OutputSizes=1
  Selector1 : Selector  IndexMode=Zero-based  InputPortWidth=POOL_SIZE  IndexOptions=Index vector (port)  Indices=[1 3]  OutputSizes=1
  Switch : Switch  Criteria=u2 ~= 0  SaturateOnIntegerOverflow=off  InputSameDT=off
  Out1 : Outport
  wires:
  Data Store Read2/1 -> Selector1/1
  Compare To Constant/1 -> AND1/2
  AND1/1 -> AND/1
  ? -> ?
  AND/1 -> Switch/2
  Switch/1 -> Data Store Write1/1, Out1/1
  PortId/1 -> Equal/1
  Equal/1 -> AND1/1
  Compare To Constant1/1 -> AND/2
  Selector1/1 -> Compare To Constant/1
  For Iterator/1 -> Selector1/2, Selector/2, Switch/1
  Data Store Read1/1 -> Compare To Constant1/1, Switch/3
  Selector/1 -> Equal/2
  Data Store Read/1 -> Selector/1

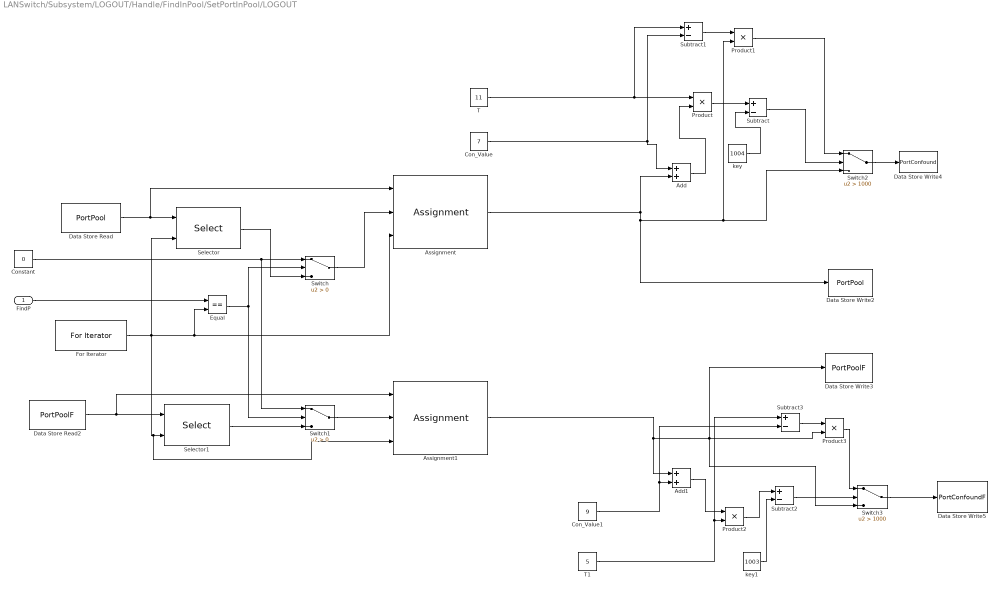
== system LANSwitch/Subsystem/LOGOUT/Handle/FindInPool/SetPortInPool/LOGOUT ==
  FindP : Inport
  Add : Sum
  Add1 : Sum
  Assignment : Assignment  IndexMode=Zero-based  DiagnosticForDimensions=Warning  IndexOptions=Index vector (port)  Indices=1  OutputSizes=1
  Assignment1 : Assignment  IndexMode=Zero-based  DiagnosticForDimensions=Warning  IndexOptions=Index vector (port)  Indices=1  OutputSizes=1
  Con_Value : Constant  Value=7  OutDataTypeStr=int32
  Con_Value1 : Constant  Value=9  OutDataTypeStr=int32
  Constant : Constant  Value=0  OutDataTypeStr=int32
  Data Store Read : DataStoreRead  DataStoreName=PortPool  IndexOptions=Index vector (dialog)  Indices=1  OutputSizes=1
  Data Store Read2 : DataStoreRead  DataStoreName=PortPoolF  IndexOptions=Index vector (dialog)  Indices=1  OutputSizes=1
  Data Store Write2 : DataStoreWrite  DataStoreName=PortPool  IndexOptions=Index vector (dialog)  Indices=1  OutputSizes=1
  Data Store Write3 : DataStoreWrite  DataStoreName=PortPoolF  IndexOptions=Index vector (dialog)  Indices=1  OutputSizes=1
  Data Store Write4 : DataStoreWrite  DataStoreName=PortConfound  IndexOptions=Index vector (dialog)  Indices=1  OutputSizes=1
  Data Store Write5 : DataStoreWrite  DataStoreName=PortConfoundF  IndexOptions=Index vector (dialog)  Indices=1  OutputSizes=1
  Equal : RelationalOperator  Operator===  OutDataTypeStr=boolean  RndMeth=Simplest  InputSameDT=off
  For Iterator : ForIterator  IterationLimit=POOL_SIZE  IndexMode=Zero-based
  Product{,1..3} (4 alike) : Product  OutDataTypeStr=int32
  Selector : Selector  IndexMode=Zero-based  InputPortWidth=POOL_SIZE  IndexOptions=Index vector (port)  Indices=[1 3]  OutputSizes=1
  Selector1 : Selector  IndexMode=Zero-based  InputPortWidth=POOL_SIZE  IndexOptions=Index vector (port)  Indices=[1 3]  OutputSizes=1
  Subtract{,1..3} (4 alike) : Sum  Inputs=+-
  Switch : Switch  Criteria=u2 > Threshold  SaturateOnIntegerOverflow=off  InputSameDT=off
  Switch1 : Switch  Criteria=u2 > Threshold  SaturateOnIntegerOverflow=off  InputSameDT=off
  Switch2 : Switch  Criteria=u2 > Threshold  Threshold=1000  SaturateOnIntegerOverflow=off  InputSameDT=off
  Switch3 : Switch  Criteria=u2 > Threshold  Threshold=1000  SaturateOnIntegerOverflow=off  InputSameDT=off
  T : Constant  Value=11  OutDataTypeStr=int32
  T1 : Constant  Value=5  OutDataTypeStr=int32
  key : Constant  Value=1004  OutDataTypeStr=int32
  key1 : Constant  Value=1003  OutDataTypeStr=int32
  wires:
  For Iterator/1 -> Assignment1/3, Selector1/2, Selector/2, Assignment/3, Equal/2
  Data Store Read/1 -> Assignment/1, Selector/1
  FindP/1 -> Equal/1
  Equal/1 -> Switch/2, Switch1/2
  Switch/1 -> Assignment/2
  Selector/1 -> Switch/3
  Constant/1 -> Switch1/1, Switch/1
  Data Store Read2/1 -> Assignment1/1, Selector1/1
  Selector1/1 -> Switch1/3
  Switch1/1 -> Assignment1/2
  Con_Value1/1 -> Subtract3/2, Add1/2
  Switch3/1 -> Data Store Write5/1
  Add/1 -> Product/2
  Con_Value/1 -> Add/1, Subtract1/2
  Assignment1/1 -> Add1/1, Product3/2, Switch3/3, Data Store Write3/1
  Subtract3/1 -> Product3/1
  Switch2/1 -> Data Store Write4/1
  Subtract2/1 -> Switch3/2
  Product3/1 -> Switch3/1
  Product2/1 -> Subtract2/1
  key1/1 -> Subtract2/2
  key/1 -> Subtract/2
  Subtract1/1 -> Product1/1
  Add1/1 -> Product2/1
  Subtract/1 -> Switch2/2
  Assignment/1 -> Product1/2, Switch2/3, Data Store Write2/1, Add/2
  T/1 -> Subtract1/1, Product/1
  T1/1 -> Subtract3/1, Product2/2
  Product/1 -> Subtract/1
  Product1/1 -> Switch2/1
